simulink model "SYSTEM"  (R2014a)
settings: Solver=ode45  StartTime=0.0  StopTime=20  RelTol=1e-3
values from neighbouring files (symbols this model uses):
  CT = inv(M)*C    [PARAMETER.m]
  KT = inv(M)*K    [PARAMETER.m]
  QT = inv(M)*Kt    [PARAMETER.m]
libraries: simulink_extras x1, simulink x1
settings Model: Creator=Administrator  LastModifiedBy=Administrator

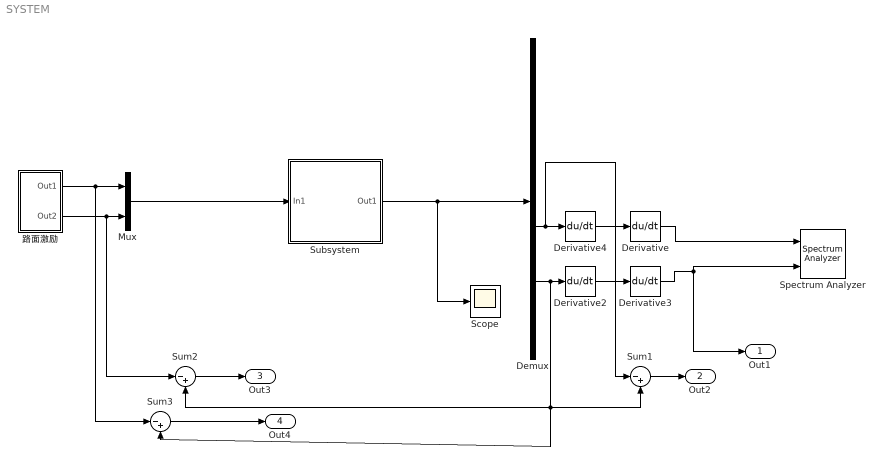
== system SYSTEM ==
  Demux : Demux  Outputs=6
  Derivative{,2..4} (4 alike) : Derivative
  Mux : Mux  Inputs=2
  Scope : Scope
  Spectrum Analyzer : simulink_extras/Additional Sinks/Spectrum Analyzer  npts=256  fftpts=256  HowOften=64  sampleT=0.1
  Subsystem : Subsystem
  Sum1 : Sum  Inputs=|-+
  Sum2 : Sum  Inputs=|-+
  Sum3 : Sum  Inputs=|-+
  "路面激励 " : Subsystem
  Out1 : Outport
  Out2 : Outport  Port=2
  Out3 : Outport  Port=3
  Out4 : Outport  Port=4
  wires:
  Demux/5 -> Sum1/2, Sum3/2, Sum2/2, Derivative2/1
  "路面激励 "/1(Out1) -> Mux/1, Sum3/1
  "路面激励 "/2(Out2) -> Mux/2, Sum2/1
  Derivative2/1 -> Derivative3/1
  Derivative3/1 -> Out1/1, Spectrum Analyzer/2
  Derivative4/1 -> Derivative/1
  Derivative/1 -> Spectrum Analyzer/1
  Demux/4 -> Sum1/1, Derivative4/1
  Sum1/1 -> Out2/1
  Sum2/1 -> Out3/1
  Sum3/1 -> Out4/1
  Subsystem/1(Out1) -> Demux/1, Scope/1
  Mux/1 -> Subsystem/1(In1)

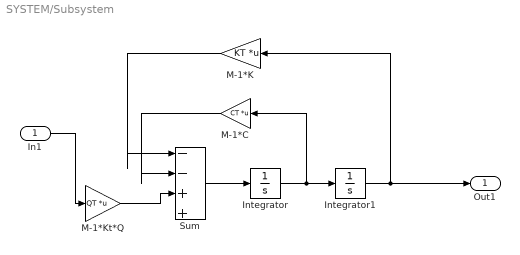
== system SYSTEM/Subsystem ==
  In1 : Inport
  Integrator : Integrator
  Integrator1 : Integrator
  M-1*C : Gain  Gain=CT  Multiplication=Matrix(K*u)
  M-1*K : Gain  Gain=KT  Multiplication=Matrix(K*u)
  M-1*Kt*Q : Gain  Gain=QT  Multiplication=Matrix(K*u)
  Sum : Sum  Inputs=|--++
  Out1 : Outport
  wires:
  M-1*Kt*Q/1 -> Sum/3
  Integrator1/1 -> Out1/1, M-1*K/1
  M-1*K/1 -> Sum/1
  Sum/1 -> Integrator/1
  M-1*C/1 -> Sum/2
  Integrator/1 -> M-1*C/1, Integrator1/1
  In1/1 -> M-1*Kt*Q/1

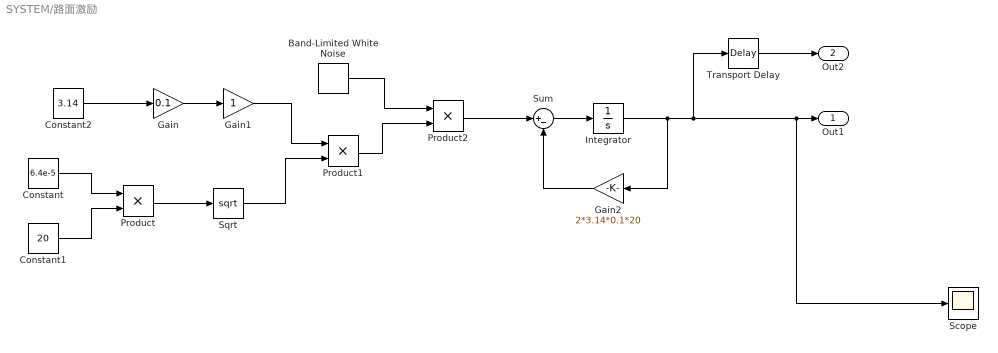
== system SYSTEM/路面激励  ==
  Band-Limited White Noise : simulink/Sources/Band-Limited White Noise  Cov=[0.1]  Ts=0.1  seed=[23341]
  Constant : Constant  Value=6.4e-5
  Constant1 : Constant  Value=20
  Constant2 : Constant  Value=3.14
  Gain : Gain  Gain=0.1
  Gain1 : Gain
  Gain2 : Gain  Gain=2*3.14*0.1*20
  Integrator : Integrator
  Product : Product
  Product1 : Product
  Product2 : Product
  Scope : Scope
  Sqrt : Sqrt  SaturateOnIntegerOverflow=on
  Sum : Sum  Inputs=|+-
  Transport Delay : TransportDelay
  Out1 : Outport
  Out2 : Outport  Port=2
  wires:
  Gain2/1 -> Sum/2
  Product/1 -> Sqrt/1
  Gain/1 -> Gain1/1
  Product1/1 -> Product2/2
  Constant/1 -> Product/1
  Sqrt/1 -> Product1/2
  Constant1/1 -> Product/2
  Constant2/1 -> Gain/1
  Band-Limited White Noise/1 -> Product2/1
  Product2/1 -> Sum/1
  Integrator/1 -> Transport Delay/1, Scope/1, Out1/1, Gain2/1
  Sum/1 -> Integrator/1
  Gain1/1 -> Product1/1
  Transport Delay/1 -> Out2/1
